simulink model "Lab_4"  (R2021b)
settings: Solver=VariableStepAuto  StartTime=0.0  StopTime=10.0  RelTol=1e-3
libraries: spsRMSLib x8, spsThreePhaseParallelRLCLoadLib x7, spsThreePhaseVIMeasurementLib x3, spsPower3phInstantaneousLib x2, spsVoltageMeasurementLib x2, spsDistributedParametersLineLib x1, spsThreePhaseSourceLib x1, spspowerguiLib x1
settings Model: Creator=coolk  LastModifiedBy=coolk

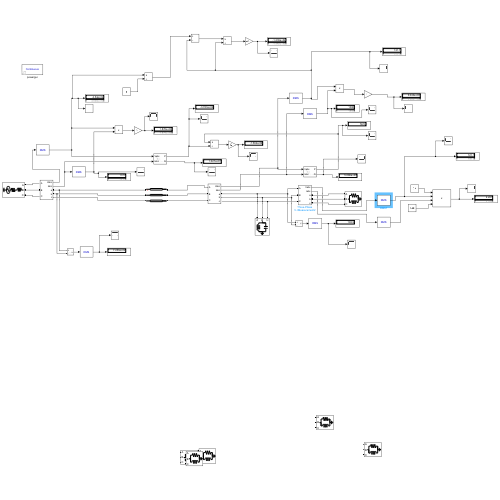
[thumbnail: Simulink's stored preview of the top-level diagram]
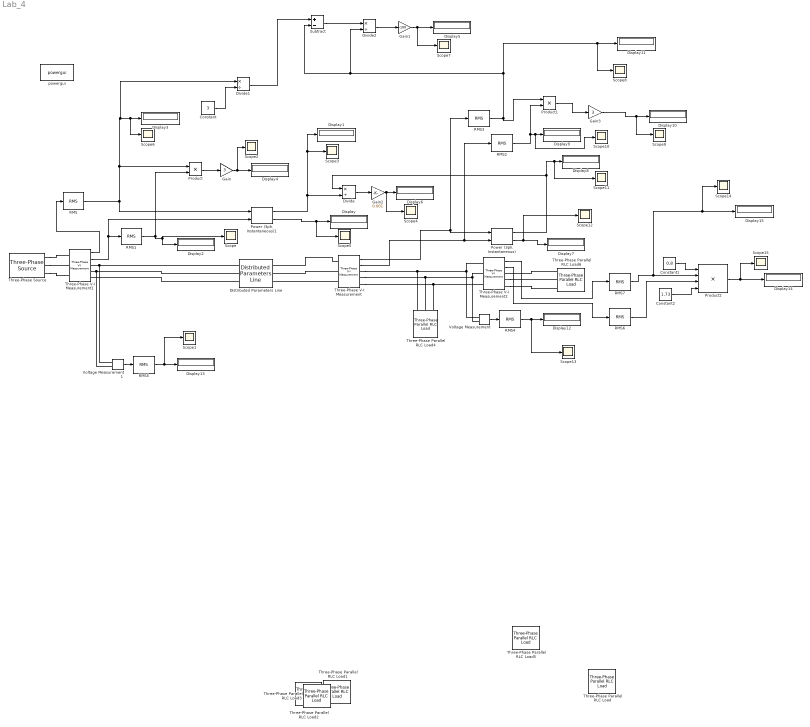
== system Lab_4 ==
  Constant : Constant  Value=3
  Constant1 : Constant  Value=0.8
  Constant2 : Constant  Value=1.73
  Display{,1..15} (16 alike) : Display
  Distributed Parameters Line : spsDistributedParametersLineLib/Distributed Parameters Line  Phases=3  Length=100  Frequency=50  Resistance=[0 0]  Inductance="[0.97e-3  0.99e-3]"  Capacitance=[11.5e-9 11.5e-9]  x1=[1.64957368524551e-10 76134.893086512 76134.8930865122;314.159265358979 314.159265358979 314.159265358979;-0.953819542280392 0.451253859539161 -1.11954246725574]  x2=[4.15044549598356e-13 201.726994437178 201.726994437178;314.159265358979 314.159265358979 314.159265358979;-1.0127527328552 0.451253858733217 -1.11954246806168]  x3=[5.55089882970319e-12 2496.39586002856 2496.39586002857;314.159265358979 314.159265358979 314.159265358979;0.504723395502222 1.91684557734072 0.346049250545825]  x4=[5.64784493161561e-12 2496.39586002968 2496.39586002969;314.159265358979 314.159265358979 314.159265358979;-2.54770235275754 -1.11926423106029 -2.69006055785518]  x5=0.00033741665637606  V1=[1.65e-10 7.613e+04 7.613e+04;314.2 314.2 314.2;-0.9538 0.4513 -1.12]  V2=[4.15e-13 201.7 201.7;314.2 314.2 314.2;-1.013 0.4513 -1.12]  I1=[5.551e-12 2496 2496;314.2 314.2 314.2;0.5047 1.917 0.346]  I2=[5.648e-12 2496 2496;314.2 314.2 314.2;-2.548 -1.119 -2.69]  nHarmo=1  Measurements=None  Decoupling=off  VsMag0=0  VrMag0=0  VsAngle0=0  VrAngle0=0  IsMag0=0  IrMag0=0  IsAngle0=0  IrAngle0=0
      settings: SourceProductBaseCode=PS
  Divide : Product  Inputs=*/
  Divide1 : Product  Inputs=*/
  Divide2 : Product  Inputs=*/
  Gain : Gain  Gain=3
  Gain1 : Gain  Gain=-100
  Gain2 : Gain  Gain=0.001
  Gain3 : Gain  Gain=3
  "Power (3ph, Instantaneous)" : spsPower3phInstantaneousLib/Power (3ph, Instantaneous)
  "Power (3ph, Instantaneous)1" : spsPower3phInstantaneousLib/Power (3ph, Instantaneous)
  Product : Product
  Product1 : Product
  Product2 : Product  Inputs=4
  RMS{,1..7} (8 alike) : spsRMSLib/RMS  TrueRMS=on  Freq=60  RMSInit=120  Ts=0
  Scope{,1..15} (16 alike) : Scope
  Subtract : Sum  Inputs=+-
  Three-Phase Parallel RLC Load{,1..3,5} (5 alike) : spsThreePhaseParallelRLCLoadLib/Three-Phase Parallel RLC Load  LConnTagsString=A|B|C  Configuration=Y (grounded)  NominalVoltage=1000  Vabc=[1e3 1e3 1e3]  Vabcp=[1e3 1e3 1e3]  NominalFrequency=60  UnbalancedPower=off  ActivePower=10e3  InductivePower=100  CapacitivePower=0  Pabc=[10e3 9e3 11e3]  QLabc=[100 90 110]  QCabc=[100 90 110]  Pabcp=[10e3 9e3 11e3]  QLabcp=[100 90 110]  QCabcp=[100 90 110]  Measurements=None  LoadType=constant Z
  Three-Phase Parallel RLC Load4 : spsThreePhaseParallelRLCLoadLib/Three-Phase Parallel RLC Load  LConnTagsString=A|B|C  Configuration=Y (grounded)  NominalVoltage=1000  Vabc=[1e3 1e3 1e3]  Vabcp=[1e3 1e3 1e3]  NominalFrequency=60  UnbalancedPower=off  ActivePower=0  InductivePower=33.75e06  CapacitivePower=33.75e06  Pabc=[10e3 9e3 11e3]  QLabc=[100 90 110]  QCabc=[100 90 110]  Pabcp=[10e3 9e3 11e3]  QLabcp=[100 90 110]  QCabcp=[100 90 110]  Measurements=None  LoadType=constant Z
  Three-Phase Parallel RLC Load6 : spsThreePhaseParallelRLCLoadLib/Three-Phase Parallel RLC Load  LConnTagsString=A|B|C  Configuration=Y (grounded)  NominalVoltage=1000  Vabc=[1e3 1e3 1e3]  Vabcp=[1e3 1e3 1e3]  NominalFrequency=60  UnbalancedPower=off  ActivePower=10e-03  InductivePower=100  CapacitivePower=0  Pabc=[10e3 9e3 11e3]  QLabc=[100 90 110]  QCabc=[100 90 110]  Pabcp=[10e3 9e3 11e3]  QLabcp=[100 90 110]  QCabcp=[100 90 110]  Measurements=None  LoadType=constant Z
  Three-Phase V-I Measurement : spsThreePhaseVIMeasurementLib/Three-Phase V-I Measurement  VoltageMeasurement=phase-to-ground  SetLabelV=off  LabelV=Vabc  Vpu=off  VpuLL=off  CurrentMeasurement=yes  SetLabelI=off  LabelI=Iabc  Ipu=off  Pbase=100e6  Vbase=500e3  OutputType=Complex  PhasorSimulation=off  PSBequivalent=0
  Three-Phase V-I Measurement1 : spsThreePhaseVIMeasurementLib/Three-Phase V-I Measurement  VoltageMeasurement=phase-to-ground  SetLabelV=off  LabelV=Vabc  Vpu=off  VpuLL=off  CurrentMeasurement=yes  SetLabelI=off  LabelI=Iabc  Ipu=off  Pbase=100e6  Vbase=500e3  OutputType=Complex  PhasorSimulation=off  PSBequivalent=0
  Three-Phase V-I Measurement2 : spsThreePhaseVIMeasurementLib/Three-Phase V-I Measurement  VoltageMeasurement=phase-to-ground  SetLabelV=off  LabelV=Vabc  Vpu=off  VpuLL=off  CurrentMeasurement=yes  SetLabelI=off  LabelI=Iabc  Ipu=off  Pbase=100e6  Vbase=500e3  OutputType=Complex  PhasorSimulation=off  PSBequivalent=0
  Three-Phase Source : spsThreePhaseSourceLib/Three-Phase Source  InternalConnection=Yg  VoltagePhases=off  Voltage=76.21e3  PhaseAngle=0  Voltage_phases=[25e3 25e3 25e3]/sqrt(3)  PhaseAngles_phases=[0 -120 +120]  Frequency=50  NonIdealSource=on  SpecifyImpedance=off  Resistance=1  Inductance=4.444e-5  ShortCircuitLevel=100e6  BaseVoltage=25e3  XRratio=7  BusType=swing  Pref=10e3  Qref=0  Prefabc=[10e3, 10e3, 10e3]  Qrefabc=[0, 0, 0]  Qmin=-inf  Qmax=inf
  Voltage Measurement : spsVoltageMeasurementLib/Voltage Measurement  PhasorSimulation=off  OutputType=Complex  PSBequivalent=0
  Voltage Measurement1 : spsVoltageMeasurementLib/Voltage Measurement  PhasorSimulation=off  OutputType=Complex  PSBequivalent=0
  powergui : spspowerguiLib/powergui  Priority=1  SimulationMode=Continuous  SampleTime=50e-6  frequency=60  Iterations=50  frequencyindice=50  Pbase=100e6  ErrMax=1e-4  UnitsV=kV  UnitsW=MW  buscounter=0  FunctionMessages=off  echomessages=off  EnableUseOfTLC=off  CurrentSourceSwitches=off  DisableSnubberDevices=off  DisableRonSwitches=off  DisableVfSwitches=off  DisplayEquations=off  AutomaticDiscreteSolvers=off  SolverType=Tustin/Backward Euler (TBE)  Interpol=off  ExternalGateDelay=off  methode=off  Ts=100  x0status=blocks  SPID=on  SwTol=0  HookPort=off  NonlinearTolerance=1e-4  nMaxIteration=100  ContinueOnMaxIteration=off  RestoreLinks=warning  ResistiveCurrentMeasurement=off  Frange=[0:2:500]  Ylog=off  Xlog=on  ShowGrid=off  save=off  variable=ZData  structure=0  ZoomFFT=off  StartTime=0.0  cycles=1  DisplayStyle=1  fundamental=60  FreqAxis=off  MaxFrequency=1000  frequencyindicesteady=1  RmsSteady=1  display=off
  wires:
  Product1/1 -> Gain3/1
  "Power (3ph, Instantaneous)1"/1 -> Scope3/1, Display1/1, Divide/2
  Gain3/1 -> Scope9/1, Display10/1
  Three-Phase V-I Measurement/2 -> RMS2/1, "Power (3ph, Instantaneous)"/2
  Divide/1 -> Gain2/1
  RMS2/1 -> Product1/2, Scope10/1, Display9/1
  Subtract/1 -> Divide2/1
  "Power (3ph, Instantaneous)"/1 -> Scope11/1, Display8/1, Divide/1
  "Power (3ph, Instantaneous)"/2 -> Scope12/1, Display7/1
  Gain/1 -> Scope2/1, Display4/1
  Gain2/1 -> Scope4/1, Display6/1
  Three-Phase V-I Measurement/1 -> RMS3/1, "Power (3ph, Instantaneous)"/1
  Product/1 -> Gain/1
  Divide1/1 -> Subtract/1
  Constant/1 -> Divide1/2
  RMS1/1 -> Display2/1, Scope/1, Product/2
  Three-Phase V-I Measurement1/1 -> RMS/1
  RMS3/1 -> Product1/1, Divide2/2, Subtract/2, Scope8/1, Display11/1
  Gain1/1 -> Scope7/1, Display5/1
  Three-Phase V-I Measurement1/2 -> RMS1/1, "Power (3ph, Instantaneous)1"/2
  Divide2/1 -> Gain1/1
  RMS/1 -> "Power (3ph, Instantaneous)1"/1, Product/1, Divide1/1, Scope6/1, Display3/1
  "Power (3ph, Instantaneous)1"/2 -> Scope5/1, Display/1
  RMS4/1 -> Scope13/1, Display12/1
  Voltage Measurement/1 -> RMS4/1
  RMS5/1 -> Scope1/1, Display13/1
  Voltage Measurement1/1 -> RMS5/1
  Three-Phase V-I Measurement2/2 -> RMS6/1
  Three-Phase V-I Measurement2/1 -> RMS7/1
  RMS6/1 -> Product2/3
  RMS7/1 -> Scope14/1, Display15/1, Product2/2
  Constant1/1 -> Product2/1
  Constant2/1 -> Product2/4
  Product2/1 -> Scope15/1, Display14/1
  connections:
  Three-Phase V-I Measurement/LConn3 -- Distributed Parameters Line/RConn3
  Three-Phase V-I Measurement/RConn1 -- Three-Phase Parallel RLC Load4/LConn1 -- Three-Phase V-I Measurement2/LConn1 -- Voltage Measurement/LConn1
  Distributed Parameters Line/LConn2 -- Voltage Measurement1/LConn2 -- Three-Phase V-I Measurement1/RConn2
  Distributed Parameters Line/LConn3 -- Three-Phase V-I Measurement1/RConn3
  Three-Phase V-I Measurement/RConn3 -- Three-Phase V-I Measurement2/LConn3 -- Three-Phase Parallel RLC Load4/LConn3
  Three-Phase Source/RConn1 -- Three-Phase V-I Measurement1/LConn1
  Three-Phase V-I Measurement/RConn2 -- Three-Phase Parallel RLC Load4/LConn2 -- Three-Phase V-I Measurement2/LConn2 -- Voltage Measurement/LConn2
  Three-Phase V-I Measurement/LConn1 -- Distributed Parameters Line/RConn1
  Three-Phase V-I Measurement/LConn2 -- Distributed Parameters Line/RConn2
  Distributed Parameters Line/LConn1 -- Voltage Measurement1/LConn1 -- Three-Phase V-I Measurement1/RConn1
  Three-Phase Source/RConn2 -- Three-Phase V-I Measurement1/LConn2
  Three-Phase Source/RConn3 -- Three-Phase V-I Measurement1/LConn3
  Three-Phase Parallel RLC Load6/LConn1 -- Three-Phase V-I Measurement2/RConn1
  Three-Phase V-I Measurement2/RConn2 -- Three-Phase Parallel RLC Load6/LConn2
  Three-Phase V-I Measurement2/RConn3 -- Three-Phase Parallel RLC Load6/LConn3
